simulink model "LookUp"  (R2020a)
settings: Solver=VariableStepAuto  StartTime=0.0  StopTime=10.0  RelTol=1e-3
values from neighbouring files (symbols this model uses):
  cx = griddata(alpha_x, mach_y, cx_values ,alpha,mach, 'v4')    [Test_Function.m]
  cz = griddata(alpha_x, mach_y, cz_values ,alpha,mach, 'v4')    [Test_Function.m]    (also in cz_inter.m = interp2(alpha_x, mach_y, cz_values, alpha, mach))
  ld_ratio = griddata(alpha_x, mach_y, LD_values ,alpha,mach, 'v4')    [Test_Function.m]    (also in lift_drag.m = griddata(alpha_x, mach_y, LD_values, alpha, mach, 'v4'))
settings Model: Creator=premk  LastModifiedBy=premk

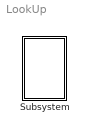
== system LookUp ==
  Subsystem : Subsystem

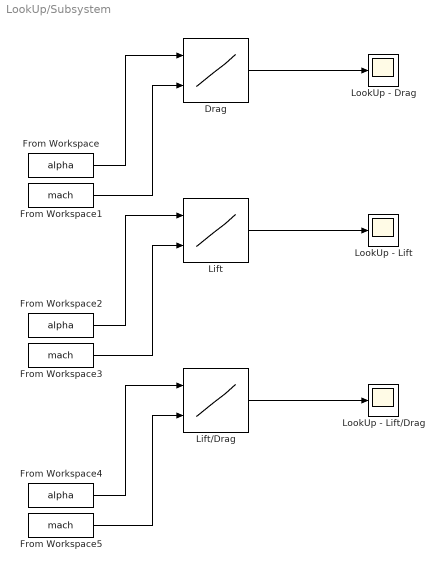
== system LookUp/Subsystem ==
  Drag : Lookup_n-D  BreakpointsSpecification=Even spacing  BreakpointsForDimension1=1  BreakpointsForDimension2=1  BreakpointsForDimension1Spacing=5  BreakpointsForDimension2Spacing=5  Table=cz  InterpMethod=Linear Lagrange  InternalRulePriority=Speed  RndMeth=Simplest  InputSameDT=on
  From Workspace : FromWorkspace  VariableName=alpha
  From Workspace1 : FromWorkspace  VariableName=mach
  From Workspace2 : FromWorkspace  VariableName=alpha
  From Workspace3 : FromWorkspace  VariableName=mach
  From Workspace4 : FromWorkspace  VariableName=alpha
  From Workspace5 : FromWorkspace  VariableName=mach
  Lift : Lookup_n-D  BreakpointsSpecification=Even spacing  BreakpointsForDimension1=1  BreakpointsForDimension2=1  BreakpointsForDimension1Spacing=5  BreakpointsForDimension2Spacing=5  Table=cx  InterpMethod=Linear Lagrange  InternalRulePriority=Speed  RndMeth=Simplest  InputSameDT=on
  Lift/Drag : Lookup_n-D  BreakpointsSpecification=Even spacing  BreakpointsForDimension1=1  BreakpointsForDimension2=1  BreakpointsForDimension1Spacing=5  BreakpointsForDimension2Spacing=5  Table=ld_ratio  InterpMethod=Linear Lagrange  InternalRulePriority=Speed  RndMeth=Simplest  InputSameDT=on
  LookUp - Drag : Scope
  LookUp - Lift : Scope
  LookUp - Lift/Drag : Scope
  wires:
  From Workspace1/1 -> Drag/2
  From Workspace/1 -> Drag/1
  From Workspace2/1 -> Lift/1
  From Workspace3/1 -> Lift/2
  Drag/1 -> LookUp - Drag/1
  Lift/1 -> LookUp - Lift/1
  From Workspace4/1 -> Lift/Drag/1
  From Workspace5/1 -> Lift/Drag/2
  Lift/Drag/1 -> LookUp - Lift/Drag/1
